simulink model "Kuka_CLIK_Model"  (R2026a)
settings: Solver=ode4  StopTime=6  FixedStep=0.002
InitFcn:
  | modelPath = fileparts(get_param(bdroot, 'FileName'));
  | addpath(modelPath);
  | q_initial = [0.05;0.35;0.15;0.75;-0.1;-0.3;0.05];
  | q_rest = zeros(7, 1);
  | p_d = [-0.00382868626777836;-0.1521848493695408;0.7458791905530762];
  | R_d = [0.5432836263310916 -0.2935452210743499 0.7865583923301243;0.5026350996614442 0.8641464937073685 -0.02467375126710217;-0.6724588150577467 0.4087567009819798 0.6170227722324836];
  | p_dot_d = zeros(3, 1);
  | omega_d = zeros(3, 1);
  | Kp_clik = 5.0 * eye(3);
  | Ko_clik = 4.0 * eye(3);
  | Kn_clik = 0.15 * eye(7);
  | lambda_clik = 1e-3;
  | clik_method = 1;
settings Model: Creator=rosales  LastModifiedBy=rosales

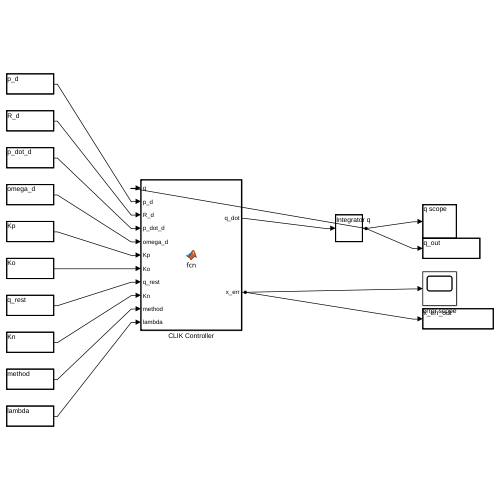
[thumbnail: Simulink's stored preview of the top-level diagram]
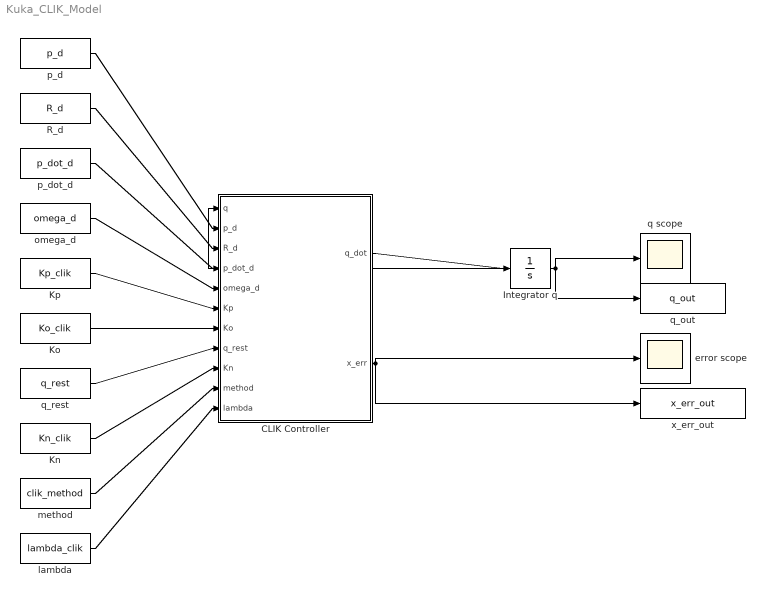
== system Kuka_CLIK_Model ==
  CLIK Controller : MATLAB Function  TreatAsAtomicUnit=on
  Integrator q : Integrator  InitialCondition=q_initial
  Kn : Constant  Value=Kn_clik
  Ko : Constant  Value=Ko_clik
  Kp : Constant  Value=Kp_clik
  R_d : Constant  Value=R_d
  error scope : Scope
  lambda : Constant  Value=lambda_clik
  method : Constant  Value=clik_method
  omega_d : Constant  Value=omega_d
  p_d : Constant  Value=p_d
  p_dot_d : Constant  Value=p_dot_d
  q scope : Scope
  q_out : ToWorkspace  VariableName=q_out  SaveFormat=Structure With Time  SampleTime=-1
  q_rest : Constant  Value=q_rest
  x_err_out : ToWorkspace  VariableName=x_err_out  SaveFormat=Structure With Time  SampleTime=-1
  wires:
  Integrator q/1 -> CLIK Controller/1(q), q scope/1, q_out/1
  p_d/1 -> CLIK Controller/2(p_d)
  R_d/1 -> CLIK Controller/3(R_d)
  p_dot_d/1 -> CLIK Controller/4(p_dot_d)
  omega_d/1 -> CLIK Controller/5(omega_d)
  Kp/1 -> CLIK Controller/6(Kp)
  Ko/1 -> CLIK Controller/7(Ko)
  q_rest/1 -> CLIK Controller/8(q_rest)
  Kn/1 -> CLIK Controller/9(Kn)
  method/1 -> CLIK Controller/10(method)
  lambda/1 -> CLIK Controller/11(lambda)
  CLIK Controller/1(q_dot) -> Integrator q/1
  CLIK Controller/2(x_err) -> error scope/1, x_err_out/1

== matlab function Kuka_CLIK_Model/CLIK Controller ==
  data: q input; q_dot output; p_d input; R_d input; p_dot_d input; omega_d input; Kp input; Ko input; q_rest input; Kn input; method input; lambda input; x_err output
function [q_dot, x_err] = fcn(q, p_d, R_d, p_dot_d, omega_d, Kp, Ko, q_rest, Kn, method, lambda)
%#codegen
[q_dot, x_err] = clik_controller(q, p_d, R_d, p_dot_d, omega_d, Kp, Ko, q_rest, Kn, method, lambda);
end
